simulink model "statespace"  (R2018b)
settings: Solver=VariableStepAuto  StartTime=0.0  StopTime=10.0  RelTol=1e-3
undefined symbols (not defined in the file or in its folder): A, B, K
settings Model: Creator=d-blo  LastModifiedBy=d-blo

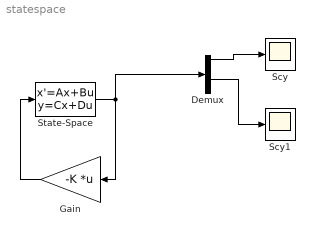
== system statespace ==
  Demux : Demux
  Gain : Gain  Gain=-K  Multiplication=Matrix(K*u)
  Scy : Scope
  Scy1 : Scope
  State-Space : StateSpace  A=A  B=B  C=eye(4)  D=zeros(4,2)  InitialCondition=[.1 0 0 0]
  wires:
  State-Space/1 -> Gain/1, Demux/1
  Gain/1 -> State-Space/1
  Demux/1 -> Scy/1
  Demux/3 -> Scy1/1
